simulink model "Seminar"  (R2022b)
settings: Solver=VariableStepAuto  StartTime=0.0  StopTime=0.15  RelTol=1e-3
values from neighbouring files (symbols this model uses):
  C = 0.0001    [seminar.m]
  L = 0.15    [seminar.m]
  R = 12    [seminar.m]
  U = 100    [seminar.m]
settings Model: Creator=manun  LastModifiedBy=manun

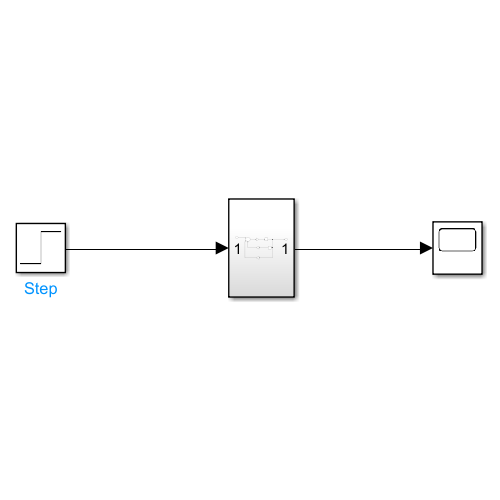
[thumbnail: Simulink's stored preview of the top-level diagram]
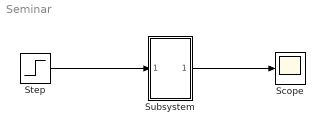
== system Seminar ==
  Scope : Scope
  Step : Step  Time=0  After=U  SampleTime=0
  Subsystem : Subsystem
  wires:
  Step/1 -> Subsystem/1(In1)
  Subsystem/1(Out1) -> Scope/1

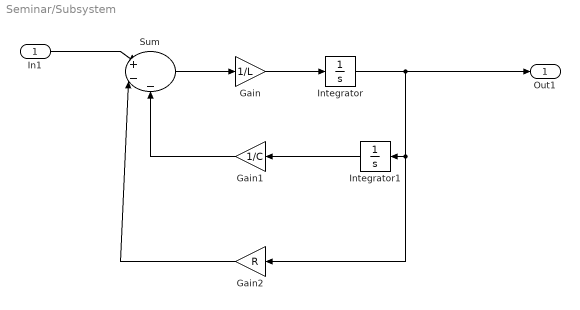
== system Seminar/Subsystem ==
  In1 : Inport
  Gain : Gain  Gain=1/L
  Gain1 : Gain  Gain=1/C
  Gain2 : Gain  Gain=R
  Integrator : Integrator
  Integrator1 : Integrator
  Sum : Sum  Inputs=|+--
  Out1 : Outport
  wires:
  Gain1/1 -> Sum/3
  Integrator/1 -> Out1/1, Gain2/1, Integrator1/1
  Gain2/1 -> Sum/2
  Sum/1 -> Gain/1
  Gain/1 -> Integrator/1
  Integrator1/1 -> Gain1/1
  In1/1 -> Sum/1
